simulink model "vehicle_longitudinal"  (R2024b)
settings: Solver=VariableStepAuto  StartTime=0.0  StopTime=200  RelTol=1e-3
undefined symbols (not defined in the file): aero, brake, downshiftRPM, magnitude, minShiftTime, pt, tire, track, upshiftRPM, veh
settings Model: Creator=nihalseth34  LastModifiedBy=nihalseth34

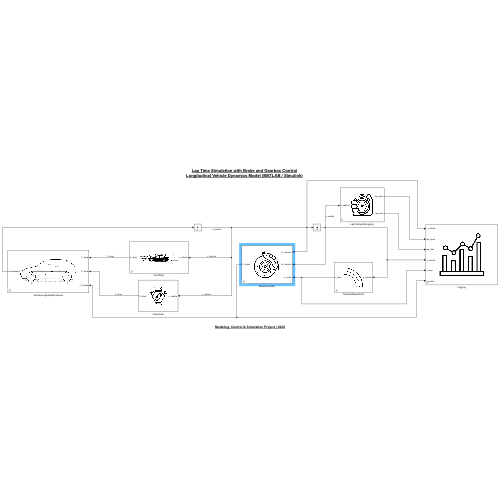
[thumbnail: Simulink's stored preview of the top-level diagram]
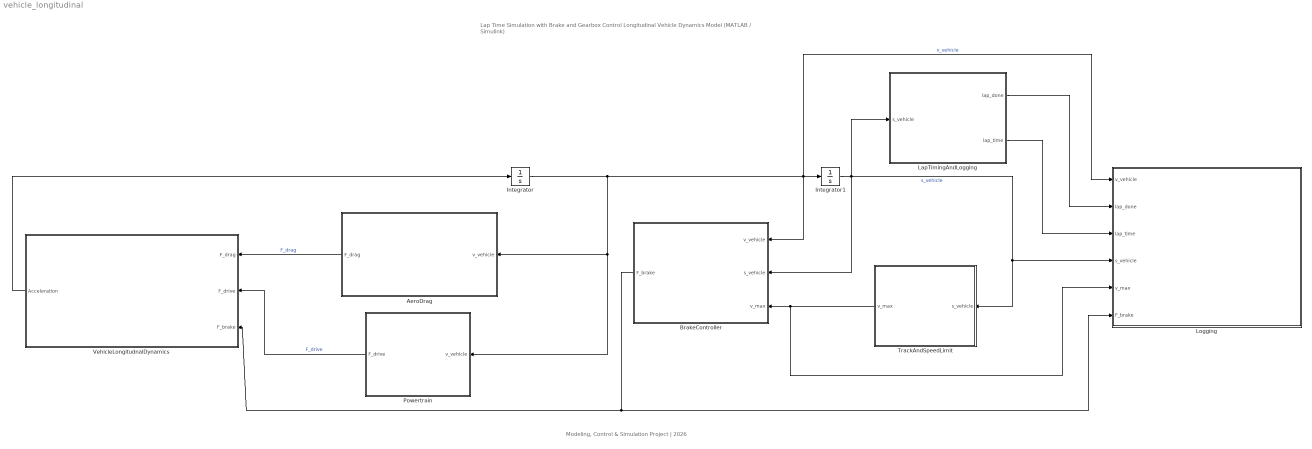
== system vehicle_longitudinal ==
  note: Modeling, Control & Simulation Project | 2026
  note: Lap Time Simulation with Brake and Gearbox Control
      | Longitudinal Vehicle Dynamics Model (MATLAB / Simulink)
  AeroDrag : Subsystem
      mask Display: image('aeroDrag.png', [0,0,0,0,80,80]);
  BrakeController : Subsystem
      mask Display: image('BrakeController.png', [0,0,0,0,70,70]);
  Integrator : Integrator
  Integrator1 : Integrator
  LapTimingAndLogging : Subsystem
      mask Display: image('LapTimingAndLogging.png', [0,0,0,0,70,70]);
  Logging : Subsystem
      mask Display: image('mask_images/Logging.png',"center");
  Powertrain : Subsystem  Description=|
      | Implements 6-speed gearbox using RPM-based hysteresis shifting.
      | Includes:
      | - Upshift logic
      | - Downshift logic
      | - Minimum shift time
      | - Rev limiter interaction
      mask Display: image('powertrain.png', [0,0,0,0,70,70]);
  TrackAndSpeedLimit : Subsystem
      mask Display: image('TrackAndSpeedLimit.png', [0,0,0,0,80,80]);
  VehicleLongitudnalDynamics : Subsystem
      mask Display: image('VehicleLongitudinalDynamics.png', [0,0,0,0,70,70]);
  wires:
  Integrator/1 -> BrakeController/1(v_vehicle), Integrator1/1, Logging/1(v_vehicle), Powertrain/1(v_vehicle), AeroDrag/1(v_vehicle)  "v_vehicle"
  Integrator1/1 -> BrakeController/2(s_vehicle), TrackAndSpeedLimit/1(s_vehicle), Logging/4(s_vehicle), LapTimingAndLogging/1(s_vehicle)  "s_vehicle"
  BrakeController/1(F_brake) -> Logging/6(F_brake), VehicleLongitudnalDynamics/3(F_brake)
  AeroDrag/1(F_drag) -> VehicleLongitudnalDynamics/1(F_drag)  "F_drag"
  VehicleLongitudnalDynamics/1(Acceleration) -> Integrator/1
  TrackAndSpeedLimit/1(v_max) -> BrakeController/3(v_max), Logging/5(v_max)
  Powertrain/1(F_drive) -> VehicleLongitudnalDynamics/2(F_drive)  "F_drive"
  LapTimingAndLogging/1(lap_done) -> Logging/2(lap_done)
  LapTimingAndLogging/2(lap_time) -> Logging/3(lap_time)

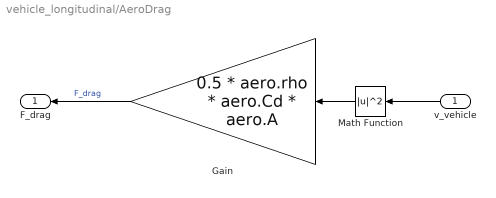
== system vehicle_longitudinal/AeroDrag ==
  v_vehicle : Inport
  Gain : Gain  Gain=0.5 * aero.rho * aero.Cd * aero.A
  Math Function : Math  Operator=magnitude^2
  F_drag : Outport
  wires:
  v_vehicle/1 -> Math Function/1
  Math Function/1 -> Gain/1
  Gain/1 -> F_drag/1  "F_drag"

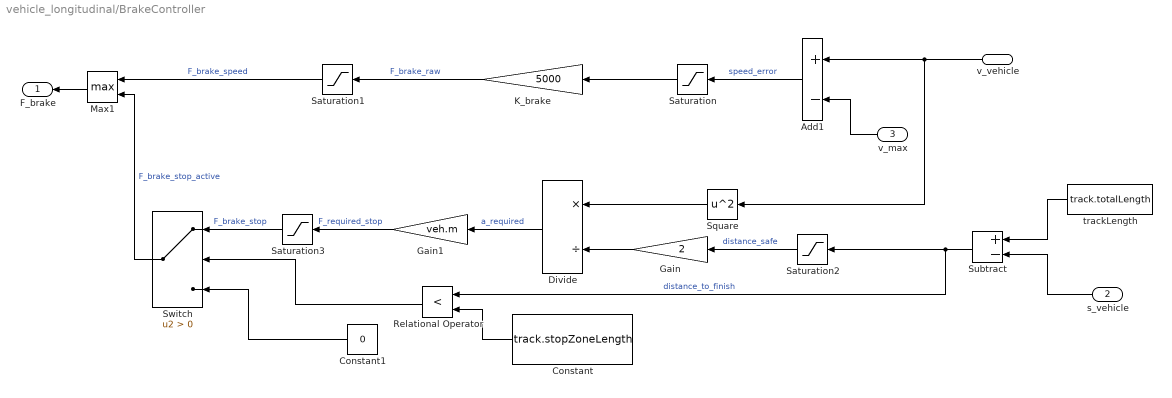
== system vehicle_longitudinal/BrakeController ==
  v_vehicle : Inport
  s_vehicle : Inport  Port=2
  v_max : Inport  Port=3
  Add1 : Sum  Inputs=+-
  Constant : Constant  Value=track.stopZoneLength
  Constant1 : Constant  Value=0
  Divide : Product  Inputs=*/
  Gain : Gain  Gain=2
  Gain1 : Gain  Gain=veh.m
  K_brake : Gain  Gain=5000
  Max1 : MinMax  Function=max  Inputs=2
  Relational Operator : RelationalOperator  Operator=<  OutDataTypeStr=boolean  RndMeth=Simplest  InputSameDT=off
  Saturation : Saturate  UpperLimit=inf  LowerLimit=0
  Saturation1 : Saturate  UpperLimit=brake.maxForce  LowerLimit=0
  Saturation2 : Saturate  UpperLimit=inf  LowerLimit=0.1
  Saturation3 : Saturate  UpperLimit=brake.maxForce  LowerLimit=0
  Square : Math  Operator=square
  Subtract : Sum  Inputs=+-
  Switch : Switch  Criteria=u2 > Threshold  SaturateOnIntegerOverflow=off  InputSameDT=off
  trackLength : Constant  Value=track.totalLength
  F_brake : Outport
  wires:
  K_brake/1 -> Saturation1/1  "F_brake_raw"
  Add1/1 -> Saturation/1  "speed_error"
  Saturation/1 -> K_brake/1
  Saturation1/1 -> Max1/1  "F_brake_speed"
  v_max/1 -> Add1/2
  trackLength/1 -> Subtract/1
  s_vehicle/1 -> Subtract/2
  Subtract/1 -> Relational Operator/1, Saturation2/1  "distance_to_finish"
  Max1/1 -> F_brake/1
  Saturation2/1 -> Gain/1  "distance_safe"
  Square/1 -> Divide/1
  Gain/1 -> Divide/2
  Divide/1 -> Gain1/1  "a_required"
  Gain1/1 -> Saturation3/1  "F_required_stop"
  Saturation3/1 -> Switch/1  "F_brake_stop"
  Constant/1 -> Relational Operator/2
  Relational Operator/1 -> Switch/2
  Constant1/1 -> Switch/3
  Switch/1 -> Max1/2  "F_brake_stop_active"
  v_vehicle/1 -> Add1/1, Square/1

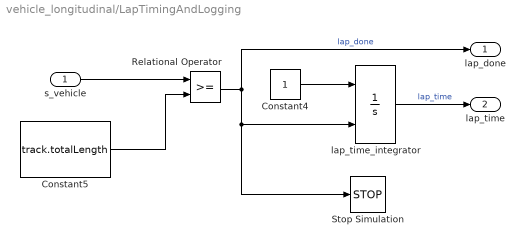
== system vehicle_longitudinal/LapTimingAndLogging ==
  s_vehicle : Inport
  Constant4 : Constant
  Constant5 : Constant  Value=track.totalLength
  Relational Operator : RelationalOperator  OutDataTypeStr=boolean  RndMeth=Simplest  InputSameDT=off
  Stop Simulation : Stop
  lap_time_integrator : Integrator  ExternalReset=rising
  lap_done : Outport
  lap_time : Outport  Port=2
  wires:
  Constant5/1 -> Relational Operator/2
  s_vehicle/1 -> Relational Operator/1
  Constant4/1 -> lap_time_integrator/1
  lap_time_integrator/1 -> lap_time/1  "lap_time"
  Relational Operator/1 -> lap_time_integrator/2, Stop Simulation/1, lap_done/1  "lap_done"

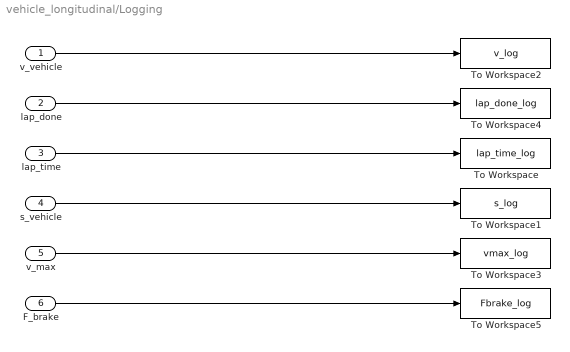
== system vehicle_longitudinal/Logging ==
  v_vehicle : Inport
  lap_done : Inport  Port=2
  lap_time : Inport  Port=3
  s_vehicle : Inport  Port=4
  v_max : Inport  Port=5
  F_brake : Inport  Port=6
  To Workspace : ToWorkspace  VariableName=lap_time_log  SampleTime=-1
  To Workspace1 : ToWorkspace  VariableName=s_log  SampleTime=-1
  To Workspace2 : ToWorkspace  VariableName=v_log  SampleTime=-1
  To Workspace3 : ToWorkspace  VariableName=vmax_log  SampleTime=-1
  To Workspace4 : ToWorkspace  VariableName=lap_done_log  SampleTime=-1
  To Workspace5 : ToWorkspace  VariableName=Fbrake_log  SampleTime=-1
  wires:
  lap_done/1 -> To Workspace4/1
  s_vehicle/1 -> To Workspace1/1
  lap_time/1 -> To Workspace/1
  v_max/1 -> To Workspace3/1
  F_brake/1 -> To Workspace5/1
  v_vehicle/1 -> To Workspace2/1

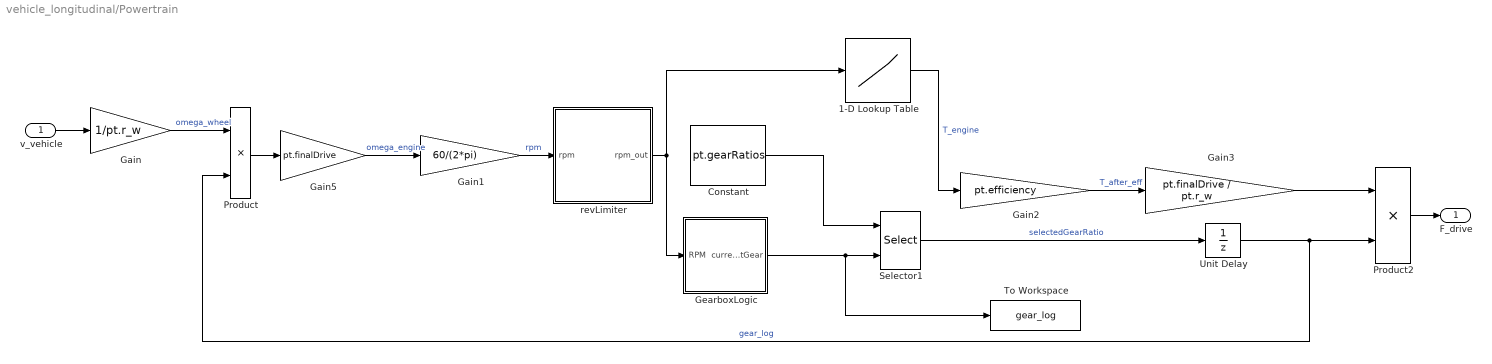
== system vehicle_longitudinal/Powertrain ==
  v_vehicle : Inport
  1-D Lookup Table : Lookup_n-D  NumberOfTableDimensions=1  BreakpointsForDimension1=pt.rpm_map  Table=pt.torque_map  InternalRulePriority=Speed  RndMeth=Simplest
  Constant : Constant  Value=pt.gearRatios
  Gain : Gain  Gain=1/pt.r_w
  Gain1 : Gain  Gain=60/(2*pi)
  Gain2 : Gain  Gain=pt.efficiency
  Gain3 : Gain  Gain=pt.finalDrive / pt.r_w
  Gain5 : Gain  Gain=pt.finalDrive
  GearboxLogic : Stateflow chart  TreatAsAtomicUnit=on
  Product : Product
  Product2 : Product
  Selector1 : Selector  InputPortWidth=6  IndexOptions=Index vector (port)  Indices=[1 3]  OutputSizes=1
  To Workspace : ToWorkspace  VariableName=gear_log  SampleTime=-1
  Unit Delay : UnitDelay  InitialCondition=pt.gearRatios(1)  SampleTime=-1  HasFrameUpgradeWarning=on
  revLimiter : Subsystem
  F_drive : Outport
  wires:
  v_vehicle/1 -> Gain/1
  Gain/1 -> Product/1  "omega_wheel"
  Product/1 -> Gain5/1
  Gain5/1 -> Gain1/1  "omega_engine"
  Gain1/1 -> revLimiter/1(rpm)  "rpm"
  1-D Lookup Table/1 -> Gain2/1  "T_engine"
  Gain2/1 -> Gain3/1  "T_after_eff"
  Constant/1 -> Selector1/1
  Selector1/1 -> Unit Delay/1  "selectedGearRatio"
  Gain3/1 -> Product2/1
  Product2/1 -> F_drive/1
  GearboxLogic/1(currentGear) -> To Workspace/1, Selector1/2
  Unit Delay/1 -> Product/2, Product2/2  "gear_log"
  revLimiter/1(rpm_out) -> GearboxLogic/1(RPM), 1-D Lookup Table/1

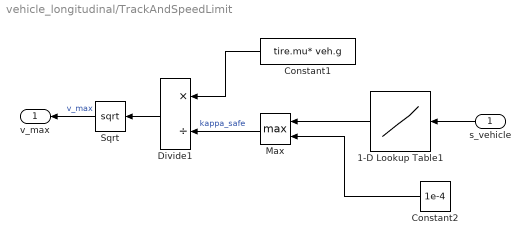
== system vehicle_longitudinal/TrackAndSpeedLimit ==
  s_vehicle : Inport
  1-D Lookup Table1 : Lookup_n-D  NumberOfTableDimensions=1  BreakpointsForDimension1=track.s  Table=track.kappa  InternalRulePriority=Speed  RndMeth=Simplest
  Constant1 : Constant  Value=tire.mu* veh.g
  Constant2 : Constant  Value=1e-4
  Divide1 : Product  Inputs=*/
  Max : MinMax  Function=max  Inputs=2
  Sqrt : Sqrt
  v_max : Outport
  wires:
  1-D Lookup Table1/1 -> Max/1
  s_vehicle/1 -> 1-D Lookup Table1/1
  Constant2/1 -> Max/2
  Constant1/1 -> Divide1/1
  Max/1 -> Divide1/2  "kappa_safe"
  Divide1/1 -> Sqrt/1
  Sqrt/1 -> v_max/1  "v_max"

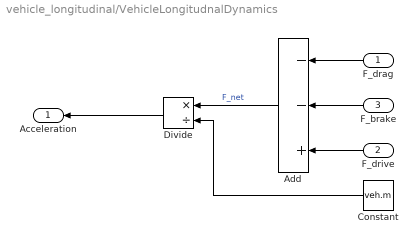
== system vehicle_longitudinal/VehicleLongitudnalDynamics ==
  F_drag : Inport
  F_drive : Inport  Port=2
  F_brake : Inport  Port=3
  Add : Sum  Inputs=--+
  Constant : Constant  Value=veh.m
  Divide : Product  Inputs=*/
  Acceleration : Outport
  wires:
  F_drag/1 -> Add/1
  Add/1 -> Divide/1  "F_net"
  Constant/1 -> Divide/2
  F_brake/1 -> Add/2
  F_drive/1 -> Add/3
  Divide/1 -> Acceleration/1

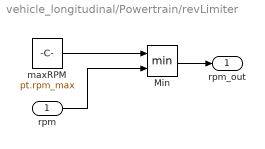
== system vehicle_longitudinal/Powertrain/revLimiter ==
  rpm : Inport
  Min : MinMax  Inputs=2
  maxRPM : Constant  Value=pt.rpm_max
  rpm_out : Outport
  wires:
  Min/1 -> rpm_out/1
  maxRPM/1 -> Min/1
  rpm/1 -> Min/2

== stateflow chart vehicle_longitudinal/Powertrain/GearboxLogic ==
  state Gear1
    entry:
    currentGear =1;
  state Gear2
    entry:
    currentGear =2;
  state Gear3
    entry:
    currentGear =3;
  state Gear4
    entry:
    currentGear =4;
  state Gear5
    entry:
    currentGear =5;
  state Gear6
    entry:
    currentGear =6;
  (default) -> Gear1
  Gear2 -> Gear1 [order 2] : [RPM <= downshiftRPM && after(minShiftTime, sec)]
  Gear1 -> Gear2 : [RPM >= upshiftRPM && after(minShiftTime, sec)]
  Gear3 -> Gear2 [order 2] : [RPM <= downshiftRPM && after(minShiftTime, sec)]
  Gear2 -> Gear3 [order 1] : [RPM >= upshiftRPM && after(minShiftTime, sec)]
  Gear4 -> Gear3 [order 2] : [RPM <= downshiftRPM && after(minShiftTime, sec)]
  Gear3 -> Gear4 [order 1] : [RPM >= upshiftRPM && after(minShiftTime, sec)]
  Gear5 -> Gear4 [order 2] : [RPM <= downshiftRPM && after(minShiftTime, sec)]
  Gear4 -> Gear5 [order 1] : [RPM >= upshiftRPM && after(minShiftTime, sec)]
  Gear6 -> Gear5 : [RPM <= downshiftRPM && after(minShiftTime, sec)]
  Gear5 -> Gear6 [order 1] : [RPM >= upshiftRPM && after(minShiftTime, sec)]
  data: RPM input double; currentGear output; upshiftRPM parameter double; downshiftRPM parameter double; minShiftTime parameter double
